simulink library "ELE819m"  (Simulink 8.1)
settings: Solver=ode45  StartTime=0.0  StopTime=10.0  RelTol=1e-3
undefined symbols (not defined in the file): Ax, Ay, Az, Kd, Kp, q1_0, q2_0, q3_0, w0, wd, wp, x0, y0, z0
settings Model: Creator=John  LastModifiedBy=John

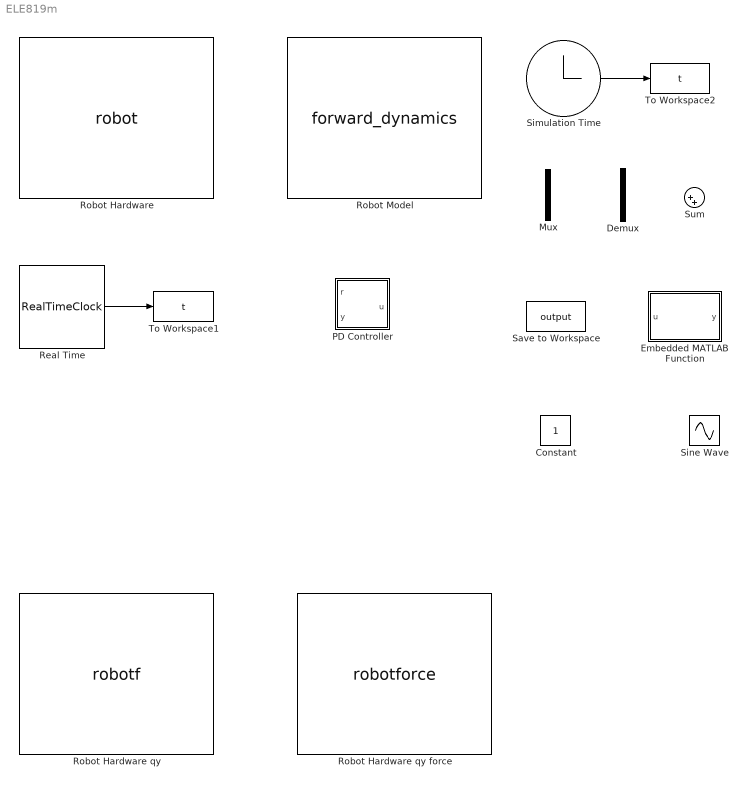
== system ELE819m ==
  Constant : Constant
  Demux : Demux  Outputs=2
  Embedded MATLAB Function : MATLAB Function  TreatAsAtomicUnit=on
  Mux : Mux  Inputs=2
  PD Controller : Subsystem  mask(PID Controller){P=Kp, D=Kd, wp=wp, wd=wd}
      mask prompts: P "Proportional:"; D "Derivative:"; wp "P gain weight"; wd "D gain weight"
      mask help:
      | Enter expressions for proportional, integral, and derivative terms.
      | P+I/s+Ds
      mask Help: This block implements a PID controller where parameters are entered for the Proportional, Integral and Derivative terms. Unmask this block to see how it works. The derivative term is implemented using a true derivative block.
      mask Display:
      | disp('PD')
      | port_label('input',1,'r');
      | port_label('input',2,'y');
  "Real Time " : S-Function  FunctionName=RealTimeClock  EnableBusSupport=off  mask(Real-Time Clock){}
      mask help: This block uses the high res clock to get real time.
      mask Display: image(imread('clock.jpg'))
  Robot Hardware : S-Function  FunctionName=robot  Parameters=Robot_Name  EnableBusSupport=off  mask{Robot_Name='Default Device'}
      mask prompts: Robot_Name "Robot Name"
      mask Display:
      | image(imread('robot.jpg'));
      | port_label('input',1,'Torque');
      | port_label('output',1,'q');
  Robot Hardware qy : S-Function  FunctionName=robotf  Parameters=Robot_Name  EnableBusSupport=off  mask{Robot_Name='Default Device'}
      mask prompts: Robot_Name "Robot Name"
      mask Display:
      | image(imread('robot.jpg'));
      | port_label('input',1,'Torque');
      | port_label('output',1,'q');
      | port_label('output',2,'y');
  Robot Hardware qy force : S-Function  FunctionName=robotforce  Parameters=Robot_Name  EnableBusSupport=off  mask{Robot_Name='Default Device'}
      mask prompts: Robot_Name "Robot Name"
      mask Display:
      | image(imread('robot.jpg'));
      | port_label('input',1,'Force');
      | port_label('output',1,'q');
      | port_label('output',2,'y');
  Robot Model : S-Function  FunctionName=forward_dynamics  Parameters=q1_0, q2_0, q3_0  EnableBusSupport=off  mask{q1_0=q1_0, q2_0=q2_0, q3_0=q3_0}
      mask prompts: q1_0 "Initial q1"; q2_0 "Initial q2"; q3_0 "Initial q3"
      mask Display:
      | image(imread('robotmodel.jpg'));
      | port_label('input',1,'Torque');
      | port_label('output',1,'q');
      | port_label('output',2,'q_dot');
  Save to Workspace : ToWorkspace  VariableName=output  SampleTime=-1
      settings: Decimation=200
  Simulation Time : Clock
      settings: Decimation=200
  Sine Wave : Sin  TimeSource=Use external signal  Amplitude="[Ax, Ay,  Az]"  Bias=[x0, y0, z0]  Frequency=[w0, w0, w0]  Phase=[0.0, pi/2, 0.0]  SampleTime=0
  Sum : Sum  Inputs=|++
  To Workspace1 : ToWorkspace  VariableName=t  SampleTime=-1
      settings: Decimation=200
  To Workspace2 : ToWorkspace  VariableName=t  SampleTime=-1
      settings: Decimation=200
  wires:
  "Real Time "/1 -> To Workspace1/1
  Simulation Time/1 -> To Workspace2/1

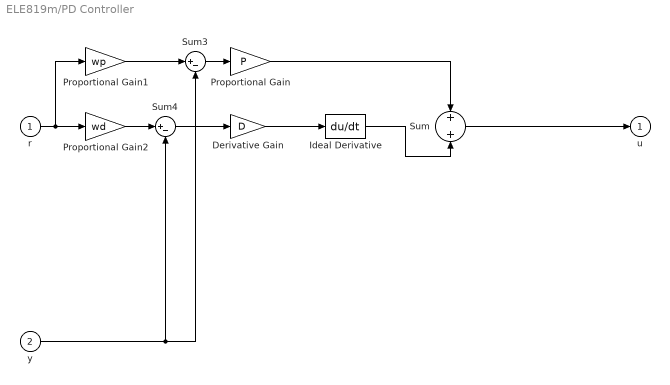
== system ELE819m/PD Controller ==
  r : Inport
  y : Inport  Port=2
  Derivative Gain : Gain  Gain=D  SaturateOnIntegerOverflow=on  OutDataTypeStr=Inherit: Same as input  ParamDataTypeStr=Inherit: Same as input
  Ideal Derivative : Derivative
  Proportional Gain : Gain  Gain=P  SaturateOnIntegerOverflow=on  OutDataTypeStr=Inherit: Same as input  ParamDataTypeStr=Inherit: Same as input
  Proportional Gain1 : Gain  Gain=wp  SaturateOnIntegerOverflow=on  OutDataTypeStr=Inherit: Same as input  ParamDataTypeStr=Inherit: Same as input
  Proportional Gain2 : Gain  Gain=wd  SaturateOnIntegerOverflow=on  OutDataTypeStr=Inherit: Same as input  ParamDataTypeStr=Inherit: Same as input
  Sum : Sum  SaturateOnIntegerOverflow=on  InputSameDT=on  OutDataTypeStr=Inherit: Same as first input
  Sum3 : Sum  Inputs=|+-
  Sum4 : Sum  Inputs=|+-
  u : Outport  InitialOutput=0
  wires:
  Sum4/1 -> Derivative Gain/1
  Sum3/1 -> Proportional Gain/1
  y/1 -> Sum3/2, Sum4/2
  r/1 -> Proportional Gain1/1, Proportional Gain2/1
  Proportional Gain1/1 -> Sum3/1
  Proportional Gain2/1 -> Sum4/1
  Derivative Gain/1 -> Ideal Derivative/1
  Sum/1 -> u/1
  Proportional Gain/1 -> Sum/1
  Ideal Derivative/1 -> Sum/2

== matlab function Embedded MATLAB Function ==
  data: u input double; y output double
function y = fcn(u)
%#eml

y = u;
